simulink model "NonLinearModelWithObserver_simulation"  (R2022a)
settings: Solver=FixedStepAuto  StartTime=0.0  StopTime=10  FixedStep=0.01  MaxStep=1e-3  MinStep=1e-5  RelTol=1e-3  EnableMultiTasking=on
values from neighbouring files (symbols this model uses):
  A = A_lin    [parameter_values.m]
  a = m1*l1^2 + m1*l2^2 + J1 + J2    (= 0.01429808)    [parameter_values.m]
  B = B_lin    [parameter_values.m]
  b = m1*l1 + m2*l2    (= 0.07644)    [parameter_values.m]
  c1 = 0.004    [parameter_values.m]
  c2 = 0.0007    [parameter_values.m]
  C_obs = [1 0 0 0; 0 0 1 0]    [parameter_values.m]
  g = 9.81    [parameter_values.m]
  J2 = 0.0001    [parameter_values.m]
  K = M_sol * inv(X_sol)    [calc_LMI_Controller.m]    (also in parameter_values.m = lqr(A,B,Q,R))
  Kb = 0.0987    [parameter_values.m]
  Kt = 0.0987    [parameter_values.m]
  L = inv(P_sol)*N_sol    [calc_LMI_Observer.m]    (also in parameter_values.m = calc_LMI_Observer(A,C_obs,10))
  Ra = 1.556    [parameter_values.m]
  theta_0 = 2*pi/180    (= 0.0349065850399)    [parameter_values.m]
  x0 = [deg2rad(0.1); 0; 0; 0]    [parameter_values.m]
  x_hat_0 = [0 0 0 0]    [parameter_values.m]
libraries: simulink_extras x1
settings Model: ExtModeTrigDuration=10  Creator=schulte  LastModifiedBy=adlipke
settings SolverCC: AlgebraicLoopSolver=TrustRegion
settings DataIOCC: ReturnWorkspaceOutputs=off
settings OptimizationCC: EnhancedBackFolding=on  PassReuseOutputArgsAs=Individual arguments  ZeroExternalMemoryAtStartup=off  ZeroInternalMemoryAtStartup=off  MaxStackSize=64  OptimizeBlockOrder=speed  DifferentSizesBufferReuse=on  OptimizationCustomize=off  EfficientTunableParamExpr=on
settings DebuggingCC: ParameterTunabilityLossMsg=error  UnconnectedInputMsg=warning  UnconnectedOutputMsg=warning  UnconnectedLineMsg=warning  SFUnexpectedBacktrackingDiag=warning  SFNoUnconditionalDefaultTransitionDiag=warning  SFMachineParentedDataDiag=warning  ArithmeticOperatorsInVariantConditions=warning
settings HardwareCC: ProdBitPerPointer=32  ProdBitPerSizeT=32  ProdBitPerPtrDiffT=32  ProdLargestAtomicInteger=Long  ProdLargestAtomicFloat=Double  ProdWordSize=32  ProdLongLongMode=on  ProdHWDeviceType=ARM Compatible->ARM Cortex
settings SFSimCC: SimUseLocalCustomCode=off  MATLABDynamicMemAlloc=off  CustomCodeUndefinedFunction=UseInterfaceOnly
settings RTWCC: SystemTargetFile=ert.tlc  HardwareBoard=STM32 Nucleo L476RG  TemplateMakefile=ert_default_tmf  RTWUseLocalCustomCode=off  Toolchain=GNU Tools for ARM Embedded Processors
settings CodeAppCC: ForceParamTrailComments=on  IgnoreCustomStorageClasses=off  OperatorAnnotations=on  SimulinkDataObjDesc=on  SFDataObjDesc=on  InsertBlockDesc=on
settings ERTTargetCC: SupportContinuousTime=on  ExtModeTransport=3  ExtModeStaticAlloc=on  ExtModeStaticAllocSize=2000  ExtModeMexFile=ext_xcp  ExtModeIntrfLevel=Level2 - Open
settings ConfigComp: CovMetricSettings=dw  CovSaveCumulativeToWorkspaceVar=on  CovSaveSingleToWorkspaceVar=on  CovExternalEMLEnable=off

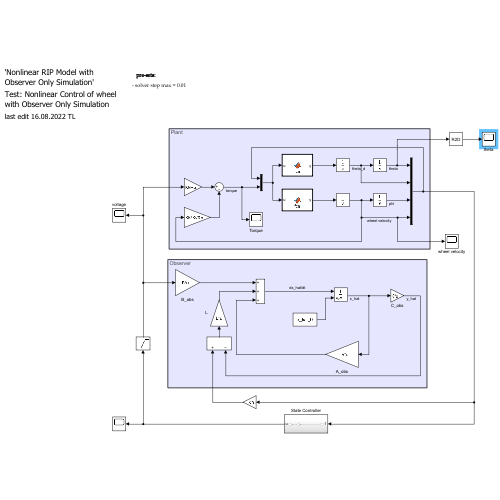
[thumbnail: Simulink's stored preview of the top-level diagram]
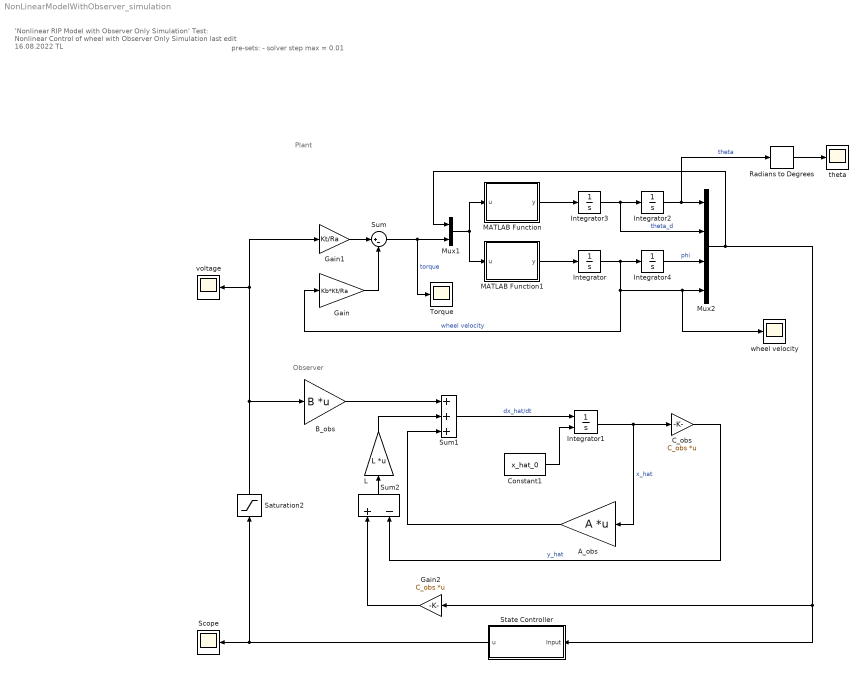
== system NonLinearModelWithObserver_simulation ==
  note: Plant
  note: Observer
  note: pre-sets:
      |
      | - solver step max = 0.01
  note: 'Nonlinear RIP Model with Observer Only Simulation'
      |
      | Test: Nonlinear Control of wheel with Observer Only Simulation
      |
      | last edit 16.08.2022 TL
  A_obs : Gain  Gain=A  Multiplication=Matrix(K*u)
  B_obs : Gain  Gain=B  Multiplication=Matrix(K*u)
  C_obs : Gain  Gain=C_obs  Multiplication=Matrix(K*u)
  Constant1 : Constant  Value=x_hat_0
  Gain : Gain  Gain=Kb*Kt/Ra
  Gain1 : Gain  Gain=Kt/Ra
  Gain2 : Gain  Gain=C_obs  Multiplication=Matrix(K*u)
  Integrator : Integrator
  Integrator1 : Integrator  InitialConditionSource=external  InitialCondition=x0
  Integrator2 : Integrator  InitialCondition=theta_0
  Integrator3 : Integrator
  Integrator4 : Integrator
  L : Gain  Gain=L  Multiplication=Matrix(K*u)
  MATLAB Function : MATLAB Function  TreatAsAtomicUnit=on
  MATLAB Function1 : MATLAB Function  TreatAsAtomicUnit=on
  Mux1 : Mux  Inputs=2
  Mux2 : Mux
  Radians to Degrees : simulink_extras/Transformations/Radians to Degrees
  Saturation2 : Saturate  UpperLimit=12  LowerLimit=-12
  Scope : Scope
  State Controller : Subsystem
  Sum : Sum  Inputs=|+-
  Sum1 : Sum  Inputs=+++
  Sum2 : Sum  Inputs=+-
  Torque : Scope
  theta : Scope
  voltage : Scope
  wheel velocity : Scope
  wires:
  A_obs/1 -> Sum1/3
  Sum2/1 -> L/1
  L/1 -> Sum1/2
  Sum1/1 -> Integrator1/1  "dx_hat/dt"
  C_obs/1 -> Sum2/2  "y_hat"
  B_obs/1 -> Sum1/1
  Constant1/1 -> Integrator1/2
  Gain2/1 -> Sum2/1
  State Controller/1(u) -> Scope/1, Saturation2/1
  Integrator1/1 -> A_obs/1, C_obs/1  "x_hat"
  Mux2/1 -> State Controller/1(Input), Gain2/1, Mux1/1
  MATLAB Function1/1(y) -> Integrator/1
  MATLAB Function/1(y) -> Integrator3/1
  Gain1/1 -> Sum/1
  Integrator4/1 -> Mux2/3  "phi"
  Integrator3/1 -> Integrator2/1, Mux2/2  "theta_d"
  Mux1/1 -> MATLAB Function1/1(u), MATLAB Function/1(u)
  Saturation2/1 -> voltage/1, Gain1/1, B_obs/1
  Gain/1 -> Sum/2
  Integrator2/1 -> Radians to Degrees/1, Mux2/1  "theta"
  Sum/1 -> Torque/1, Mux1/2  "torque"
  Integrator/1 -> wheel velocity/1, Mux2/4, Gain/1, Integrator4/1  "wheel velocity"
  Radians to Degrees/1 -> theta/1

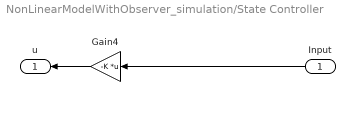
== system NonLinearModelWithObserver_simulation/State Controller ==
  Input : Inport
  Gain4 : Gain  Gain=-K  Multiplication=Matrix(K*u)
  u : Outport
  wires:
  Gain4/1 -> u/1
  Input/1 -> Gain4/1

== matlab function NonLinearModelWithObserver_simulation/MATLAB Function1 ==
  data: u input size=5; y output; a parameter; b parameter; g parameter; c1 parameter; c2 parameter; J2 parameter
function y = fcn(u, a, b, g, c1, c2, J2)

y = (a*u(5)/J2+c1*u(2)-b*g*sin(u(1))-a*c2*u(4)/J2)/(a-J2);

== matlab function NonLinearModelWithObserver_simulation/MATLAB Function ==
  data: u input size=5; y output; a parameter; b parameter; g parameter; c1 parameter; c2 parameter; J2 parameter
function y = fcn(u, a, b, g, c1, c2, J2)

y = (b*g*sin(u(1))-c1*u(2)+c2*u(4)-u(5))/(a-J2);
